simulink model "Copy_of_model_1st"  (R2020b)
settings: Solver=FixedStepAuto  StartTime=0.0  StopTime=250  FixedStep=0.1  RelTol=1e-3
libraries: simulink_extras x4, fuzblock x1
settings Model: Creator=凌寒  LastModifiedBy=凌寒

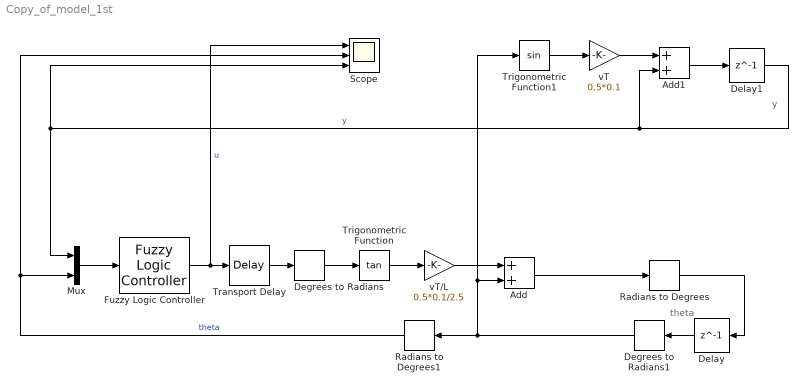
== system Copy_of_model_1st ==
  note: theta
  note: y
  Add : Sum
  Add1 : Sum
  Degrees to Radians : simulink_extras/Transformations/Degrees to Radians
  Degrees to Radians1 : simulink_extras/Transformations/Degrees to Radians
  Delay : Delay  DelayLength=1  InitialCondition=-140  StateName=theta
  Delay1 : Delay  DelayLength=1  InitialCondition=30  StateName=theta
  Fuzzy Logic Controller : fuzblock/Fuzzy Logic  Controller  FIS='myfuzzy.fis'  OutputSampleNumber=101  DataType=double  FuzzifiedInputs=off  RuleFiringStrengths=off  RuleOutputs=off  AggregatedOutputs=off  SimulateUsing=Interpreted execution  OutOfRangeInputValueMessage=warning  NoRuleFiredMessage=warning  EmptyOutputFuzzySetMessage=warning
  Mux : Mux  Inputs=2
  Radians to Degrees : simulink_extras/Transformations/Radians to Degrees
  Radians to Degrees1 : simulink_extras/Transformations/Radians to Degrees
  Scope : Scope  NumInputPorts=3
  Transport Delay : TransportDelay
  Trigonometric Function : Trigonometry  Operator=tan
  Trigonometric Function1 : Trigonometry
  vT : Gain  Gain=0.5*0.1
  vT/L : Gain  Gain=0.5*0.1/2.5
  wires:
  Trigonometric Function/1 -> vT/L/1
  Mux/1 -> Fuzzy Logic Controller/1
  Add/1 -> Radians to Degrees/1
  Trigonometric Function1/1 -> vT/1
  vT/1 -> Add1/1
  Delay1/1 -> Add1/2, Mux/1, Scope/3  "y"
  Fuzzy Logic Controller/1 -> Scope/1, Transport Delay/1  "u"
  Transport Delay/1 -> Degrees to Radians/1
  vT/L/1 -> Add/1
  Radians to Degrees/1 -> Delay/1
  Delay/1 -> Degrees to Radians1/1
  Degrees to Radians1/1 -> Add/2, Trigonometric Function1/1, Radians to Degrees1/1
  Degrees to Radians/1 -> Trigonometric Function/1
  Add1/1 -> Delay1/1
  Radians to Degrees1/1 -> Mux/2, Scope/2  "theta"
